simulink model "simulation_file"  (R2023b)
settings: Solver=FixedStepAuto  StartTime=0.0  StopTime=16  FixedStep=0.001  RelTol=1e-3
InitFcn:
  | importfrankaEmikaPanda
values from neighbouring files (symbols this model uses):
  d_influence = 0.06    [distance_with_linesegments_test.m]    (also in importfrankaEmikaPanda.m; matlab_obstacle_avoidance.m = 0.04)
  d_stop = 0.02    [distance_with_linesegments_test.m]    (also in importfrankaEmikaPanda.m; matlab_obstacle_avoidance.m = 0.01)
  Gripper_orientation = [-pi/4 0 0]    [importfrankaEmikaPanda.m]
  Gripper_position = [0 0 0.103399]    [importfrankaEmikaPanda.m]
  Homejointpositions = [0 ,0, 0, -pi/2, 0, pi/2, pi/4]    [importfrankaEmikaPanda.m]
  jointMaxValues = [2.8973, 1.7628, 2.8973, -0.0698, 2.8973, 3.7525, 2.8973]    [importfrankaEmikaPanda.m]
  jointMinValues = [-2.8973, -1.7628, -2.8973, -3.0718, -2.8973, 0.6500, -2.8973]    [importfrankaEmikaPanda.m]
  jointvelMaxValues = [2.1750 2.1750 2.1750 2.1750 2.6100 2.6100 2.6100]    [importfrankaEmikaPanda.m]
  jointvelMinValues = [-2.1750 -2.1750 -2.1750 -2.1750 -2.6100 -2.6100 -2.6100]    [importfrankaEmikaPanda.m]
  m = sqrt(det(JJt))    [computeManipulabilityJacobian.m]
  maxWaypoints = 20    [createWaypointData.m]    (also in importfrankaEmikaPanda.m)
  mdhparams = [ ... (first row only)    [importfrankaEmikaPanda.m]
  obstacle_sphere_1 = struct(     'type', OBSTACLE_SPHERE,      'center', [0, 0.20, 0.8],      'dimensions', [0.1, 0.1, 0.1],      'orientation', [1, 0, 0, 0],      'axis', 0  )    [importfrankaEmikaPanda.m]    (also in matlab_obstacle_avoidance.m = struct(     'type', OBSTACLE_SPHERE,      'center', [0.5545,)
  orientations = [0     0    0 ... (first row only)    [createWaypointData.m]    (also in importfrankaEmikaPanda.m = orientations'; matlab_obstacle_avoidance.m = orientations')
  ts = 0.01    [createWaypointData.m]    (also in importfrankaEmikaPanda.m = 0.001; matlab_obstacle_avoidance.m = 0.001)
  waypointAccels = zeros(size(waypointVels))    [createWaypointData.m]    (also in importfrankaEmikaPanda.m; matlab_obstacle_avoidance.m)
  waypoints = toolPositionHome' +              [0 0 0 ; 0 0 0 ; 0 0 0 ; 0 0 0 ; 0 0 0]'    [createWaypointData.m]    (also in importfrankaEmikaPanda.m = waypoints'; matlab_obstacle_avoidance.m = waypoints')
  waypointTimes = 0:4:16    [createWaypointData.m]    (also in importfrankaEmikaPanda.m; matlab_obstacle_avoidance.m)
  waypointVels = 0.1 *[ 0  0  0 ... (first row only)    [createWaypointData.m]    (also in importfrankaEmikaPanda.m; matlab_obstacle_avoidance.m)
  X = X + v0(1)    [plotCylinder.m]    (also in plotCylinder_foranimation.m)
  Y = Y + v0(2)    [plotCylinder.m]    (also in plotCylinder_foranimation.m)
  Z = Z + v0(3)    [plotCylinder.m]    (also in plotCylinder_foranimation.m)
undefined symbols (not defined in the file or in its folder): diff
libraries: sm_lib x98, nesl_utility x15, robotmaniplib x11, trajExampleUtils x9, robotcorelib x7
(part 1 of 4)
settings Model: Creator=shobhit  LastModifiedBy=shobhit
settings ModelReferenceCC: EnableRefExpFcnMdlSchedulingChecks=on

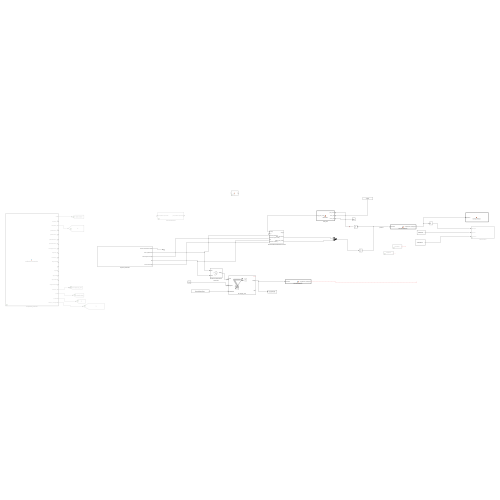
[thumbnail: Simulink's stored preview of the top-level diagram]
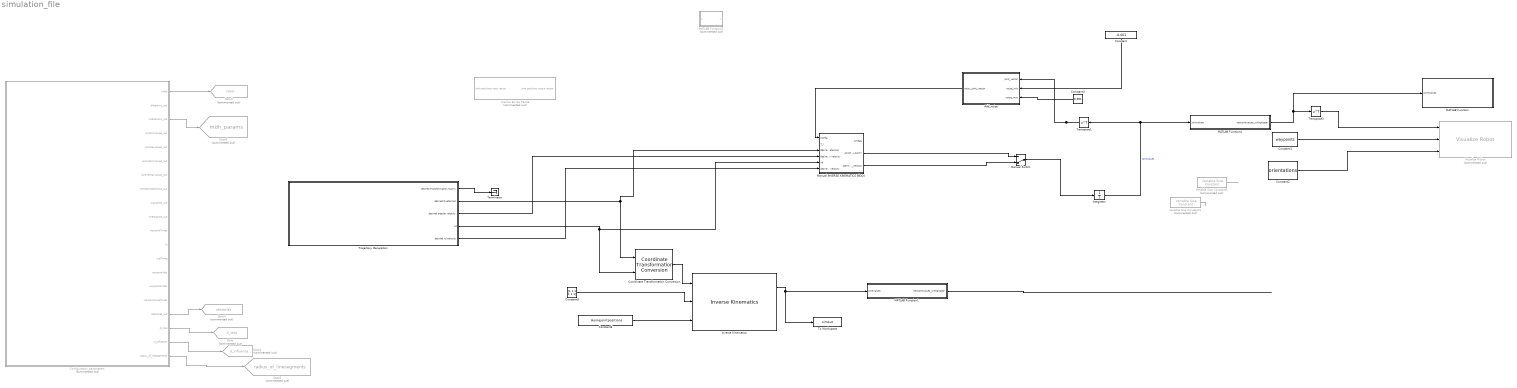
== system simulation_file ==
  Add_noise : MATLAB Function  TreatAsAtomicUnit=on
  Configuration_parameters : MATLAB Function  Commented=on  TreatAsAtomicUnit=on  SystemSampleTime=0.001
  Constant : Constant  Value=-0.001
  Constant1 : Constant  Value=waypoints  SampleTime=ts
  Constant2 : Constant  Value=orientations  VectorParams1D=off  SampleTime=ts
  Constant3 : Constant  Value=0.001
  Constant5 : Constant  Value=[1 1 1 1 1 1]
  Constant6 : Constant  Value=Homejointpositions  VectorParams1D=off
  Coordinate Transformation Conversion : robotcorelib/Coordinate Transformation Conversion  InputRepresentation=Quaternion  InputEulerSequence=ZYX  ShowTrVecInputPort=on  OutputRepresentation=Homogeneous Transformation  OutputEulerSequence=ZYX  ShowTrVecOutputPort=on  SimulateUsing=Interpreted execution
  Franka Emika Panda : Subsystem  Commented=on
  Goto : Goto  Commented=on  GotoTag=d_stop  TagVisibility=global
  Goto1 : Goto  Commented=on  GotoTag=d_influence  TagVisibility=global
  Goto2 : Goto  Commented=on  GotoTag=radius_of_linesegments  TagVisibility=global
  Goto3 : Goto  Commented=on  GotoTag=robot  TagVisibility=global
  Goto4 : Goto  Commented=on  GotoTag=obstacles  TagVisibility=global
  Goto5 : Goto  Commented=on  GotoTag=mdh_params  TagVisibility=global
  Integrator : Integrator  InitialCondition=[0 ;0; 0; -pi/2; 0; pi/2; pi/4]
  Inverse Kinematics : robotmaniplib/Inverse Kinematics  RigidBodyTree=frankarobot_mdh  EndEffector=Gripper_TCP  ShowInfo=on  SolverName=BFGS Gradient Projection  EnforceJointLimits=on  MaxIterations=1500  MaxTime=10  GradientTolerance=1e-7  SolutionTolerance=1e-6  StepTolerance=1e-14  ErrorChangeTolerance=1e-12  UseErrorDamping=on  DampingBias=0.0025  SimulateUsing=Interpreted execution
  MATLAB Function : MATLAB Function  TreatAsAtomicUnit=on
  MATLAB Function1 : MATLAB Function  TreatAsAtomicUnit=on
  MATLAB Function4 : MATLAB Function  TreatAsAtomicUnit=on
  MATLAB Function5 : MATLAB Function  Commented=on  TreatAsAtomicUnit=on
  Manual INVERSE KINEMATICS BlOCK : Subsystem
  Manual Switch : ManualSwitch  CurrentSetting=0
  Terminator : Terminator
  To Workspace : ToWorkspace  VariableName=simout  SaveFormat=Timeseries  SampleTime=-1
  Trajectory Generation : Subsystem
  Transpose1 : Math  Operator=transpose
  Transpose3 : Math  Operator=transpose
  Variable Size Constant1 : trajExampleUtils/Variable Size Constant  Commented=on  val=waypoints  maxSize=[3,maxWaypoints]  Ts=ts
  Variable Size Constant6 : trajExampleUtils/Variable Size Constant  Commented=on  val=orientations  maxSize=[3,maxWaypoints]  Ts=ts
  Visualize Robot : trajExampleUtils/Visualize Robot  Commented=on  rbtName=frankarobot  eeName=Gripper_TCP  numJoints=9  maxPts=5  plotMode=Trajectory
  wires:
  Trajectory Generation/4(xd) -> Manual INVERSE KINEMATICS BlOCK/5(xd), Coordinate Transformation Conversion/2
  Trajectory Generation/1(desired Transformation matrix) -> Terminator/1
  Variable Size Constant1/1 -> ?
  Variable Size Constant6/1 -> ?
  Constant1/1 -> Visualize Robot/2
  Constant2/1 -> Visualize Robot/3
  MATLAB Function4/1(newjointvalues_withgripper) -> MATLAB Function/1(jointValues), Transpose3/1
  Trajectory Generation/2(desired Quaternion) -> Coordinate Transformation Conversion/1, Manual INVERSE KINEMATICS BlOCK/3(desired Quaternion)
  Coordinate Transformation Conversion/1 -> Inverse Kinematics/1
  Constant5/1 -> Inverse Kinematics/2
  Constant6/1 -> Inverse Kinematics/3
  Inverse Kinematics/1 -> MATLAB Function1/1(jointvalues), To Workspace/1
  MATLAB Function1/1(newjointvalues_withgripper) -> ?
  Transpose3/1 -> Visualize Robot/1
  Integrator/1 -> Transpose1/1, MATLAB Function4/1(jointvalues)  "jointvalues"
  Trajectory Generation/3(desired angular velocity) -> Manual INVERSE KINEMATICS BlOCK/4(desired angular velocity)
  Trajectory Generation/5(desired xd velocity) -> Manual INVERSE KINEMATICS BlOCK/6(desired xd velocity)
  Manual INVERSE KINEMATICS BlOCK/2(JOINT_VELOCITY) -> Manual Switch/1
  Manual Switch/1 -> Integrator/1
  Manual INVERSE KINEMATICS BlOCK/3(optimal_joint_velocity) -> Manual Switch/2
  Constant/1 -> Add_noise/2(noise_min)
  Constant3/1 -> Add_noise/3(noise_max)
  Add_noise/1(noisy_joint_vector) -> Manual INVERSE KINEMATICS BlOCK/1(Config)
  Transpose1/1 -> Add_noise/1(joint_vector)
  Configuration_parameters/18(d_stop) -> Goto/1
  Configuration_parameters/19(d_influence) -> Goto1/1
  Configuration_parameters/20(radius_of_linesegments) -> Goto2/1
  Configuration_parameters/1(robot) -> Goto3/1
  Configuration_parameters/17(obstacles_out) -> Goto4/1
  Configuration_parameters/3(mdhparams_out) -> Goto5/1

== system simulation_file/Franka Emika Panda ==
  joint positions input vector : Inport
  Demux : Demux  Outputs=7
  Franka_Robot : Subsystem
  Joint positions vector from sensor : Mux  Inputs=7
  joint positions output vector : Outport
  wires:
  Franka_Robot/4(Output3) -> Joint positions vector from sensor/4
  Joint positions vector from sensor/1 -> joint positions output vector/1
  Franka_Robot/1(Output) -> Joint positions vector from sensor/1
  Demux/6 -> Franka_Robot/6(Input5)
  joint positions input vector/1 -> Demux/1
  Demux/5 -> Franka_Robot/5(Input4)
  Demux/3 -> Franka_Robot/3(Input2)
  Franka_Robot/6(Output5) -> Joint positions vector from sensor/6
  Demux/4 -> Franka_Robot/4(Input3)
  Demux/7 -> Franka_Robot/7(Input6)
  Franka_Robot/2(Output1) -> Joint positions vector from sensor/2
  Franka_Robot/3(Output2) -> Joint positions vector from sensor/3
  Demux/1 -> Franka_Robot/1(Input)
  Franka_Robot/7(Output6) -> Joint positions vector from sensor/7
  Demux/2 -> Franka_Robot/2(Input1)
  Franka_Robot/5(Output4) -> Joint positions vector from sensor/5

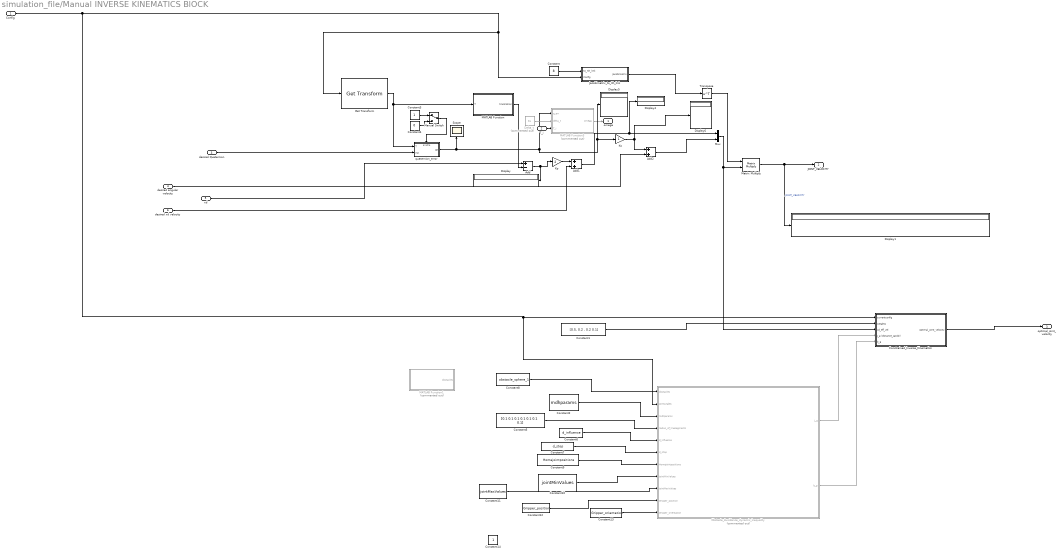
== system simulation_file/Manual INVERSE KINEMATICS BlOCK ==
  Config : Inport
  T_i : Inport  Port=2
  desired Quaternion : Inport  Port=3
  desired angular velocity : Inport  Port=4
  xd : Inport  Port=5
  desired xd velocity : Inport  Port=6
  Add : Sum  Inputs=+-
  Add1 : Sum
  Add2 : Sum
  Constant : Constant  Value=8
  Constant1 : Constant  Value=[0.5, 0.2 , 0.2 0.1]
  Constant10 : Constant  Value=jointMinValues  VectorParams1D=off
  Constant11 : Constant  Value=jointMaxValues  VectorParams1D=off
  Constant12 : Constant  Value=Gripper_position  VectorParams1D=off
  Constant13 : Constant  Value=Gripper_orientation  VectorParams1D=off
  Constant14 : Constant
  Constant2 : Constant  Value=mdhparams  VectorParams1D=off
  Constant3 : Constant
  Constant4 : Constant  Value=0
  Constant5 : Constant  Value=[0.1 0.1 0.1 0.1 0.1 0.1 0.1]  VectorParams1D=off
  Constant6 : Constant  Value=d_influence  VectorParams1D=off
  Constant7 : Constant  Value=d_stop  VectorParams1D=off
  Constant8 : Constant  Value=obstacle_sphere_1  VectorParams1D=off  OutDataTypeStr=Bus: slBus1
  Constant9 : Constant  Value=Homejointpositions  VectorParams1D=off
  Constrained_Inverse_Kinematics : Subsystem
  Delta_t : Constant  Commented=on  Value=ts
  Display{,1,4..6} (5 alike) : Display
  Get Transform : robotmaniplib/Get Transform  RigidBodyTree=frankarobot_mdh  SourceBody=Gripper_TCP  TargetBody=base  SimulateUsing=Interpreted execution
  Jacobimatrix_to_ith_link : Subsystem
  Ko : Gain
  Kp : Gain  Gain=2
  MATLAB Function : MATLAB Function  TreatAsAtomicUnit=on
  MATLAB Function1 : MATLAB Function  Commented=on  TreatAsAtomicUnit=on
  MATLAB Function3 : MATLAB Function  Commented=on  TreatAsAtomicUnit=on
  Manual Switch : ManualSwitch
  Matrix Multiply : Product  Multiplication=Matrix(*)
  Mux : Mux  Inputs=2
  Obstacle_Avoidance_dynamic_inequality : MATLAB Function  Commented=on  TreatAsAtomicUnit=on
  Scope : Scope
  Transpose : Math  Operator=transpose
  quaternion_error : Subsystem
  omega : Outport
  JOINT_VELOCITY : Outport  Port=2
  optimal_joint_velocity : Outport  Port=3
  wires:
  MATLAB Function/1(translation) -> Add/2
  desired Quaternion/1 -> quaternion_error/2(In2)
  Manual Switch/1 -> quaternion_error/Enable
  MATLAB Function3/1(omega) -> omega/1
  Kp/1 -> Add1/1
  quaternion_error/1(qe) -> Ko/1, Display5/1, MATLAB Function3/1(q_err), Scope/1
  Add/1 -> Display/1, Kp/1
  Mux/1 -> Constrained_Inverse_Kinematics/3(xd_eff_vel), Matrix Multiply/2
  Constant4/1 -> Manual Switch/2
  Constant3/1 -> Manual Switch/1
  Ko/1 -> Display6/1, Add2/1
  Add2/1 -> Mux/2
  Jacobimatrix_to_ith_link/1(Jacobimatrix) -> Transpose/1
  Matrix Multiply/1 -> JOINT_VELOCITY/1, Display1/1  "JOINT_VELOCITY"
  Get Transform/1 -> quaternion_error/1(T), MATLAB Function/1(T)
  desired angular velocity/1 -> Add2/2
  xd/1 -> Add/1
  Constant/1 -> Jacobimatrix_to_ith_link/1(to_ith_link)
  desired xd velocity/1 -> Add1/2
  Transpose/1 -> Matrix Multiply/1
  Add1/1 -> Display4/1, Mux/1
  T_i/1 -> MATLAB Function3/3(T_i)
  Delta_t/1 -> MATLAB Function3/2(delta_t)
  Constant1/1 -> Constrained_Inverse_Kinematics/2(weights)
  Config/1 -> Obstacle_Avoidance_dynamic_inequality/2(jointAngles), Constrained_Inverse_Kinematics/1(currentconfig), Jacobimatrix_to_ith_link/2(Config), Get Transform/1
  Constrained_Inverse_Kinematics/1(optimal_joint_velocity) -> optimal_joint_velocity/1
  Obstacle_Avoidance_dynamic_inequality/1(J_g) -> Constrained_Inverse_Kinematics/4(J_g (distance_Jacobi))
  Obstacle_Avoidance_dynamic_inequality/2(b_g) -> Constrained_Inverse_Kinematics/5("b_g ")
  Constant2/1 -> Obstacle_Avoidance_dynamic_inequality/3(mdhparams)
  Constant5/1 -> Obstacle_Avoidance_dynamic_inequality/4(radius_of_linesegments)
  Constant6/1 -> Obstacle_Avoidance_dynamic_inequality/5(d_influence)
  Constant7/1 -> Obstacle_Avoidance_dynamic_inequality/6(d_stop)
  Constant8/1 -> Obstacle_Avoidance_dynamic_inequality/1(obstacles)
  Constant9/1 -> Obstacle_Avoidance_dynamic_inequality/7(Homejointpositions)
  Constant10/1 -> Obstacle_Avoidance_dynamic_inequality/8(jointMinValues)
  Constant11/1 -> Obstacle_Avoidance_dynamic_inequality/9(jointMaxValues)
  Constant12/1 -> Obstacle_Avoidance_dynamic_inequality/10(Gripper_position)
  Constant13/1 -> Obstacle_Avoidance_dynamic_inequality/11(Gripper_orientation)

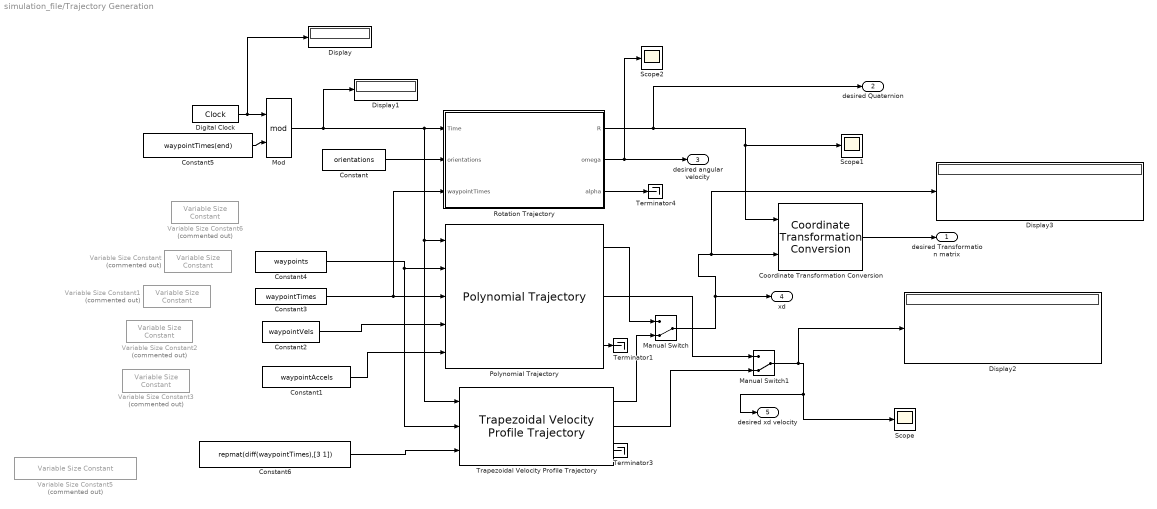
== system simulation_file/Trajectory Generation ==
  Constant : Constant  Value=orientations  SampleTime=ts
  Constant1 : Constant  Value=waypointAccels  SampleTime=ts
  Constant2 : Constant  Value=waypointVels  SampleTime=ts
  Constant3 : Constant  Value=waypointTimes  SampleTime=ts
  Constant4 : Constant  Value=waypoints  SampleTime=ts
  Constant5 : Constant  Value=waypointTimes(end)
  Constant6 : Constant  Value=repmat(diff(waypointTimes),[3 1])  SampleTime=ts
  Coordinate Transformation Conversion : robotcorelib/Coordinate Transformation Conversion  InputRepresentation=Quaternion  InputEulerSequence=ZYX  ShowTrVecInputPort=on  OutputRepresentation=Homogeneous Transformation  OutputEulerSequence=ZYX  ShowTrVecOutputPort=on  SimulateUsing=Interpreted execution
  Digital Clock : DigitalClock  SampleTime=ts
  Display{,1..3} (4 alike) : Display
  Manual Switch : ManualSwitch  CurrentSetting=0
  Manual Switch1 : ManualSwitch  CurrentSetting=0
  Mod : Math  Operator=mod  SignedPower=on
  Polynomial Trajectory : robotcorelib/Polynomial Trajectory  WaypointSource=External  Waypoints=[ 0, 2, 1, 5, 0; -1, 3, 1, 4, 4 ]  TimePoints=[ 0, 1, 2, 3, 4 ]  TimeInterval=[ 1, 4 ]  Method=Quintic Polynomial  ParameterSource=External  VelocityBoundaryCondition=zeros( 2, 5 )  AccelerationBoundaryCondition=zeros( 2, 5 )  SimulateUsing=Interpreted execution
  Rotation Trajectory : Subsystem
  Scope : Scope
  Scope1 : Scope
  Scope2 : Scope
  Terminator1 : Terminator
  Terminator3 : Terminator
  Terminator4 : Terminator
  Trapezoidal Velocity Profile Trajectory : robotcorelib/Trapezoidal Velocity Profile Trajectory  WaypointSource=External  Waypoints=[ 0, -0.5, -1; 0, 0.5, 1 ]  NumParams=1  Parameter1=End Time  Parameter2=End Time  ParameterSource=External  PeakVelocity=[ 1; 1; 1 ]  Acceleration=[ 1; 2 ]  EndTime=[ 1; 1; 1 ]  AccelTime=[ 1; 2 ]  SimulateUsing=Interpreted execution
  Variable Size Constant : trajExampleUtils/Variable Size Constant  Commented=on  val=waypoints  maxSize=[3,maxWaypoints]  Ts=ts
  Variable Size Constant1 : trajExampleUtils/Variable Size Constant  Commented=on  val=waypointTimes  maxSize=[1,maxWaypoints]  Ts=ts
  Variable Size Constant2 : trajExampleUtils/Variable Size Constant  Commented=on  val=waypointVels  maxSize=[3,maxWaypoints]  Ts=ts
  Variable Size Constant3 : trajExampleUtils/Variable Size Constant  Commented=on  val=waypointAccels  maxSize=[3,maxWaypoints]  Ts=ts
  Variable Size Constant5 : trajExampleUtils/Variable Size Constant  Commented=on  val=repmat(diff(waypointTimes),[3 1])  maxSize=[3,maxWaypoints-1]  Ts=ts
  Variable Size Constant6 : trajExampleUtils/Variable Size Constant  Commented=on  val=orientations  maxSize=[3,maxWaypoints]  Ts=ts
  desired Transformation matrix : Outport
  desired Quaternion : Outport  Port=2
  desired angular velocity : Outport  Port=3
  xd : Outport  Port=4
  desired xd velocity : Outport  Port=5
  wires:
  Trapezoidal Velocity Profile Trajectory/3 -> Terminator3/1
  Constant2/1 -> Polynomial Trajectory/4
  Constant4/1 -> Trapezoidal Velocity Profile Trajectory/2, Polynomial Trajectory/2
  Constant6/1 -> Trapezoidal Velocity Profile Trajectory/3
  Polynomial Trajectory/3 -> Terminator1/1
  Polynomial Trajectory/1 -> Manual Switch/1
  Trapezoidal Velocity Profile Trajectory/1 -> Manual Switch/2
  Constant/1 -> Rotation Trajectory/2(orientations)
  Trapezoidal Velocity Profile Trajectory/2 -> Manual Switch1/2
  Mod/1 -> Display1/1, Rotation Trajectory/1(Time), Trapezoidal Velocity Profile Trajectory/1, Polynomial Trajectory/1
  Constant1/1 -> Polynomial Trajectory/5
  Coordinate Transformation Conversion/1 -> desired Transformation matrix/1
  Constant3/1 -> Rotation Trajectory/3(waypointTimes), Polynomial Trajectory/3
  Rotation Trajectory/1(R) -> desired Quaternion/1, Coordinate Transformation Conversion/1, Scope1/1
  Constant5/1 -> Mod/2
  Digital Clock/1 -> Display/1, Mod/1
  Polynomial Trajectory/2 -> Manual Switch1/1
  Manual Switch/1 -> Display3/1, Coordinate Transformation Conversion/2, xd/1
  Rotation Trajectory/2(omega) -> Scope2/1, desired angular velocity/1
  Rotation Trajectory/3(alpha) -> Terminator4/1
  Manual Switch1/1 -> Display2/1, Scope/1, desired xd velocity/1

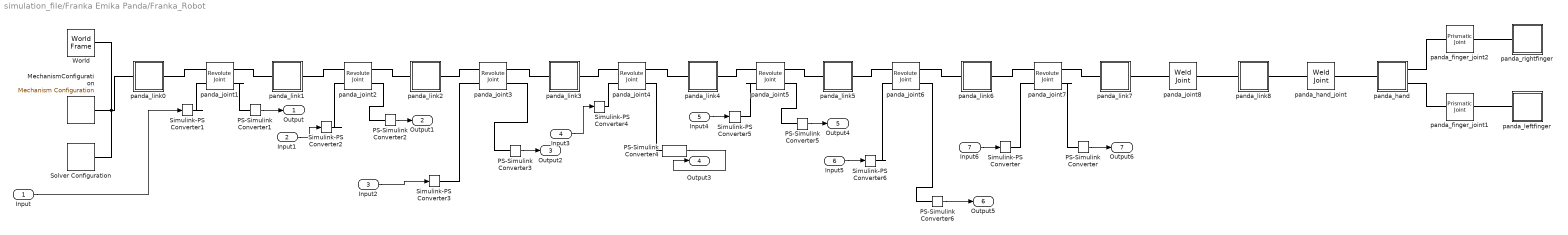
== system simulation_file/Franka Emika Panda/Franka_Robot ==
  Input : Inport
  Input1 : Inport  Port=2
  Input2 : Inport  Port=3
  Input3 : Inport  Port=4
  Input4 : Inport  Port=5
  Input5 : Inport  Port=6
  Input6 : Inport  Port=7
  MechanismConfiguration : sm_lib/Utilities/Mechanism Configuration  UniformGravity=Constant  GravityVector=[0, 0, 0]  GravityVectorUnits=m/s^2  LinearizationDelta=0.001  JointModeTransitionNonlinearIterations=2
  PS-Simulink Converter{,1..6} (7 alike) : nesl_utility/PS-Simulink Converter  PhysicalDomain=network_engine_domain  SubClassName=ps_output  LeftPortType=input  RightPortType=output  PseudoPeriodic=off  Frequencies=[]  VectorFormat=inherit  Unit=inherit  AffineConversion=off
  Simulink-PS Converter{,1,3..6} (6 alike) : nesl_utility/Simulink-PS Converter  PhysicalDomain=network_engine_domain  SubClassName=ps_input  LeftPortType=input  RightPortType=output  PseudoPeriodic=off  Frequencies=[]  NoiseDistribution=none  NoiseParameters=[]  Unit=1  AffineConversion=off  FilteringAndDerivatives=provide  SimscapeFilterOrder=1  InputFilterTimeConstant=0.001  UdotUserProvided=0
  Simulink-PS Converter2 : nesl_utility/Simulink-PS Converter  PhysicalDomain=network_engine_domain  SubClassName=ps_input  LeftPortType=input  RightPortType=output  PseudoPeriodic=off  Frequencies=[]  NoiseDistribution=none  NoiseParameters=[]  Unit=1  AffineConversion=off  FilteringAndDerivatives=filter  SimscapeFilterOrder=1  InputFilterTimeConstant=0.001  UdotUserProvided=0
  Solver Configuration : nesl_utility/Solver Configuration  PhysicalDomain=network_engine_domain  SubClassName=solver  LeftPortType=input  RightPortType=generic  Tones=[]  Harmonics=[]  SimulateNoise=off  Profile=off  UseLocalSampling=off  EnableSwitchedLinearOptims=on  FrequencyDomain=off  UseCCode=off  RelTol=0.001  AbsTol=0.001  MinStep=1e-09  ToWorkspace=off  RevertToSquareIcSolve=off  NumHomotopyIterations=100  PhasorMode=off  PhasorModeNumHarmonics=1  ConsistencySolver=NEWTON_XTOL_AFTER_FTOL  IndexReductionMethod=DerivativeReplacement  DoDC=off  ResidualTolerance=1e-09  ConsistencyTolSource=GLOBAL  ConsistencyAbsTol=0.001  ConsistencyRelTol=0.001  ConsistencyTolFactor=0.001  UseLocalSolver=off  LocalSolverChoice=NE_BACKWARD_EULER_ADVANCER  ResolveIndetEquations=on  FunctionEvalNumThread=1  LocalSolverSampleTime=0.001  DoFixedCost=off  MaxNonlinIter=3  MaxModeIter=2  ComputeImpulses=off  ImpulseIterations=2  LinearAlgebra=auto  LinearAlgebraNumThread=0  EquationFormulation=NE_TIME_EF  DelaysMemoryBudget=1024  AutomaticFiltering=on  FilteringTimeConstant=0.001  PartitionStorageMethod=AS_NEEDED  PartitionMemoryBudget=1024  PartitionMethod=ROBUST  MultibodyUseLocalSolver=off  MultibodyLocalSolverChoice=ODE1  MultibodyLocalSolverSampleTime=0.001
  World : sm_lib/Frames and Transforms/World Frame
  panda_finger_joint1 : sm_lib/Joints/Prismatic Joint  JointMode=Normal  SenseConstraintForce=off  SenseConstraintForceX=off  SenseConstraintForceY=off  SenseConstraintForceZ=off  SenseConstraintTorque=off  SenseConstraintTorqueX=off  SenseConstraintTorqueY=off  SenseConstraintTorqueZ=off  SenseTotalForce=off  SenseTotalForceX=off  SenseTotalForceY=off  SenseTotalForceZ=off  SenseTotalTorque=off  SenseTotalTorqueX=off  SenseTotalTorqueY=off  SenseTotalTorqueZ=off  CompositeWrenchDir=FollowerOnBase  CompositeWrenchFrame=BaseFrame  EquilibriumPosition=0  EquilibriumPositionUnits=m  SpringStiffness=0  SpringStiffnessUnits=N/m  DampingCoefficient=0  DampingCoefficientUnits=kg/s  TorqueActuationMode=NoTorque  MotionActuationMode=ComputedMotion  SensePosition=off  SenseVelocity=off  SenseAcceleration=off  SenseTorqueForce=off  SenseLowerLimitTorqueForce=off  SenseUpperLimitTorqueForce=off  LowerLimitSpecify=on  LowerLimitBound=0  LowerLimitBoundUnits=m  LowerLimitStiffness=1e6  LowerLimitStiffnessUnits=N/m  LowerLimitDamping=1e3  LowerLimitDampingUnits=N/(m/s)  LowerLimitTransitionRegionWidth=1e-4  LowerLimitTransitionRegionWidthUnits=m  UpperLimitSpecify=on  UpperLimitBound=0.04  UpperLimitBoundUnits=m  UpperLimitStiffness=1e6  UpperLimitStiffnessUnits=N/m  UpperLimitDamping=1e3  UpperLimitDampingUnits=N/(m/s)  UpperLimitTransitionRegionWidth=1e-4  UpperLimitTransitionRegionWidthUnits=m  PositionTargetSpecify=on  PositionTargetPriority=High  PositionTargetValue=0  PositionTargetValueUnits=m  VelocityTargetSpecify=off  VelocityTargetPriority=High  VelocityTargetValue=0  VelocityTargetValueUnits=m/s
  panda_finger_joint2 : sm_lib/Joints/Prismatic Joint  JointMode=Normal  SenseConstraintForce=off  SenseConstraintForceX=off  SenseConstraintForceY=off  SenseConstraintForceZ=off  SenseConstraintTorque=off  SenseConstraintTorqueX=off  SenseConstraintTorqueY=off  SenseConstraintTorqueZ=off  SenseTotalForce=off  SenseTotalForceX=off  SenseTotalForceY=off  SenseTotalForceZ=off  SenseTotalTorque=off  SenseTotalTorqueX=off  SenseTotalTorqueY=off  SenseTotalTorqueZ=off  CompositeWrenchDir=FollowerOnBase  CompositeWrenchFrame=BaseFrame  EquilibriumPosition=0  EquilibriumPositionUnits=m  SpringStiffness=0  SpringStiffnessUnits=N/m  DampingCoefficient=0  DampingCoefficientUnits=kg/s  TorqueActuationMode=NoTorque  MotionActuationMode=ComputedMotion  SensePosition=off  SenseVelocity=off  SenseAcceleration=off  SenseTorqueForce=off  SenseLowerLimitTorqueForce=off  SenseUpperLimitTorqueForce=off  LowerLimitSpecify=on  LowerLimitBound=0  LowerLimitBoundUnits=m  LowerLimitStiffness=1e6  LowerLimitStiffnessUnits=N/m  LowerLimitDamping=1e3  LowerLimitDampingUnits=N/(m/s)  LowerLimitTransitionRegionWidth=1e-4  LowerLimitTransitionRegionWidthUnits=m  UpperLimitSpecify=on  UpperLimitBound=0.04  UpperLimitBoundUnits=m  UpperLimitStiffness=1e6  UpperLimitStiffnessUnits=N/m  UpperLimitDamping=1e3  UpperLimitDampingUnits=N/(m/s)  UpperLimitTransitionRegionWidth=1e-4  UpperLimitTransitionRegionWidthUnits=m  PositionTargetSpecify=on  PositionTargetPriority=High  PositionTargetValue=0  PositionTargetValueUnits=m  VelocityTargetSpecify=off  VelocityTargetPriority=High  VelocityTargetValue=0  VelocityTargetValueUnits=m/s
  panda_hand : Subsystem
  panda_hand_joint : sm_lib/Joints/Weld Joint  JointMode=Normal  SenseConstraintForce=off  SenseConstraintForceX=off  SenseConstraintForceY=off  SenseConstraintForceZ=off  SenseConstraintTorque=off  SenseConstraintTorqueX=off  SenseConstraintTorqueY=off  SenseConstraintTorqueZ=off  SenseTotalForce=off  SenseTotalForceX=off  SenseTotalForceY=off  SenseTotalForceZ=off  SenseTotalTorque=off  SenseTotalTorqueX=off  SenseTotalTorqueY=off  SenseTotalTorqueZ=off  CompositeWrenchDir=FollowerOnBase  CompositeWrenchFrame=BaseFrame
  panda_joint{1,3,5,7} (4 alike) : sm_lib/Joints/Revolute Joint  JointMode=Normal  SenseConstraintForce=off  SenseConstraintForceX=off  SenseConstraintForceY=off  SenseConstraintForceZ=off  SenseConstraintTorque=off  SenseConstraintTorqueX=off  SenseConstraintTorqueY=off  SenseConstraintTorqueZ=off  SenseTotalForce=off  SenseTotalForceX=off  SenseTotalForceY=off  SenseTotalForceZ=off  SenseTotalTorque=off  SenseTotalTorqueX=off  SenseTotalTorqueY=off  SenseTotalTorqueZ=off  CompositeWrenchDir=FollowerOnBase  CompositeWrenchFrame=BaseFrame  EquilibriumPosition=0  EquilibriumPositionUnits=deg  SpringStiffness=0  SpringStiffnessUnits=N*m/deg  DampingCoefficient=0  DampingCoefficientUnits=kg*m^2/(rad*s)  TorqueActuationMode=NoTorque  MotionActuationMode=InputMotion  SensePosition=on  SenseVelocity=off  SenseAcceleration=off  SenseTorqueForce=off  SenseLowerLimitTorqueForce=off  SenseUpperLimitTorqueForce=off  LowerLimitSpecify=on  LowerLimitBound=-2.8973  LowerLimitBoundUnits=rad  LowerLimitStiffness=1e4  LowerLimitStiffnessUnits=N*m/deg  LowerLimitDamping=10  LowerLimitDampingUnits=N*m/(deg/s)  LowerLimitTransitionRegionWidth=0.1  LowerLimitTransitionRegionWidthUnits=deg  UpperLimitSpecify=on  UpperLimitBound=2.8973  UpperLimitBoundUnits=rad  UpperLimitStiffness=1e4  UpperLimitStiffnessUnits=N*m/deg  UpperLimitDamping=10  UpperLimitDampingUnits=N*m/(deg/s)  UpperLimitTransitionRegionWidth=0.1  UpperLimitTransitionRegionWidthUnits=deg  PositionTargetSpecify=off  PositionTargetPriority=High  PositionTargetValue=0  PositionTargetValueUnits=rad  VelocityTargetSpecify=off  VelocityTargetPriority=High  VelocityTargetValue=0  VelocityTargetValueUnits=deg/s
  panda_joint2 : sm_lib/Joints/Revolute Joint  JointMode=Normal  SenseConstraintForce=off  SenseConstraintForceX=off  SenseConstraintForceY=off  SenseConstraintForceZ=off  SenseConstraintTorque=off  SenseConstraintTorqueX=off  SenseConstraintTorqueY=off  SenseConstraintTorqueZ=off  SenseTotalForce=off  SenseTotalForceX=off  SenseTotalForceY=off  SenseTotalForceZ=off  SenseTotalTorque=off  SenseTotalTorqueX=off  SenseTotalTorqueY=off  SenseTotalTorqueZ=off  CompositeWrenchDir=FollowerOnBase  CompositeWrenchFrame=BaseFrame  EquilibriumPosition=0  EquilibriumPositionUnits=deg  SpringStiffness=0  SpringStiffnessUnits=N*m/deg  DampingCoefficient=0  DampingCoefficientUnits=kg*m^2/(rad*s)  TorqueActuationMode=NoTorque  MotionActuationMode=InputMotion  SensePosition=on  SenseVelocity=off  SenseAcceleration=off  SenseTorqueForce=off  SenseLowerLimitTorqueForce=off  SenseUpperLimitTorqueForce=off  LowerLimitSpecify=on  LowerLimitBound=-1.7628  LowerLimitBoundUnits=rad  LowerLimitStiffness=1e4  LowerLimitStiffnessUnits=N*m/deg  LowerLimitDamping=10  LowerLimitDampingUnits=N*m/(deg/s)  LowerLimitTransitionRegionWidth=0.1  LowerLimitTransitionRegionWidthUnits=deg  UpperLimitSpecify=on  UpperLimitBound=1.7628  UpperLimitBoundUnits=rad  UpperLimitStiffness=1e4  UpperLimitStiffnessUnits=N*m/deg  UpperLimitDamping=10  UpperLimitDampingUnits=N*m/(deg/s)  UpperLimitTransitionRegionWidth=0.1  UpperLimitTransitionRegionWidthUnits=deg  PositionTargetSpecify=off  PositionTargetPriority=High  PositionTargetValue=-1.5708  PositionTargetValueUnits=rad  VelocityTargetSpecify=off  VelocityTargetPriority=High  VelocityTargetValue=0  VelocityTargetValueUnits=deg/s
  panda_joint4 : sm_lib/Joints/Revolute Joint  JointMode=Normal  SenseConstraintForce=off  SenseConstraintForceX=off  SenseConstraintForceY=off  SenseConstraintForceZ=off  SenseConstraintTorque=off  SenseConstraintTorqueX=off  SenseConstraintTorqueY=off  SenseConstraintTorqueZ=off  SenseTotalForce=off  SenseTotalForceX=off  SenseTotalForceY=off  SenseTotalForceZ=off  SenseTotalTorque=off  SenseTotalTorqueX=off  SenseTotalTorqueY=off  SenseTotalTorqueZ=off  CompositeWrenchDir=FollowerOnBase  CompositeWrenchFrame=BaseFrame  EquilibriumPosition=0  EquilibriumPositionUnits=deg  SpringStiffness=0  SpringStiffnessUnits=N*m/deg  DampingCoefficient=0  DampingCoefficientUnits=kg*m^2/(rad*s)  TorqueActuationMode=NoTorque  MotionActuationMode=InputMotion  SensePosition=on  SenseVelocity=off  SenseAcceleration=off  SenseTorqueForce=off  SenseLowerLimitTorqueForce=off  SenseUpperLimitTorqueForce=off  LowerLimitSpecify=on  LowerLimitBound=-3.0718  LowerLimitBoundUnits=rad  LowerLimitStiffness=1e4  LowerLimitStiffnessUnits=N*m/deg  LowerLimitDamping=10  LowerLimitDampingUnits=N*m/(deg/s)  LowerLimitTransitionRegionWidth=0.1  LowerLimitTransitionRegionWidthUnits=deg  UpperLimitSpecify=on  UpperLimitBound=-0.0698  UpperLimitBoundUnits=rad  UpperLimitStiffness=1e4  UpperLimitStiffnessUnits=N*m/deg  UpperLimitDamping=10  UpperLimitDampingUnits=N*m/(deg/s)  UpperLimitTransitionRegionWidth=0.1  UpperLimitTransitionRegionWidthUnits=deg  PositionTargetSpecify=off  PositionTargetPriority=High  PositionTargetValue=0  PositionTargetValueUnits=rad  VelocityTargetSpecify=off  VelocityTargetPriority=High  VelocityTargetValue=0  VelocityTargetValueUnits=deg/s
  panda_joint6 : sm_lib/Joints/Revolute Joint  JointMode=Normal  SenseConstraintForce=off  SenseConstraintForceX=off  SenseConstraintForceY=off  SenseConstraintForceZ=off  SenseConstraintTorque=off  SenseConstraintTorqueX=off  SenseConstraintTorqueY=off  SenseConstraintTorqueZ=off  SenseTotalForce=off  SenseTotalForceX=off  SenseTotalForceY=off  SenseTotalForceZ=off  SenseTotalTorque=off  SenseTotalTorqueX=off  SenseTotalTorqueY=off  SenseTotalTorqueZ=off  CompositeWrenchDir=FollowerOnBase  CompositeWrenchFrame=BaseFrame  EquilibriumPosition=0  EquilibriumPositionUnits=deg  SpringStiffness=0  SpringStiffnessUnits=N*m/deg  DampingCoefficient=0  DampingCoefficientUnits=kg*m^2/(rad*s)  TorqueActuationMode=NoTorque  MotionActuationMode=InputMotion  SensePosition=on  SenseVelocity=off  SenseAcceleration=off  SenseTorqueForce=off  SenseLowerLimitTorqueForce=off  SenseUpperLimitTorqueForce=off  LowerLimitSpecify=on  LowerLimitBound=-0.0175  LowerLimitBoundUnits=rad  LowerLimitStiffness=1e4  LowerLimitStiffnessUnits=N*m/deg  LowerLimitDamping=10  LowerLimitDampingUnits=N*m/(deg/s)  LowerLimitTransitionRegionWidth=0.1  LowerLimitTransitionRegionWidthUnits=deg  UpperLimitSpecify=on  UpperLimitBound=3.7525  UpperLimitBoundUnits=rad  UpperLimitStiffness=1e4  UpperLimitStiffnessUnits=N*m/deg  UpperLimitDamping=10  UpperLimitDampingUnits=N*m/(deg/s)  UpperLimitTransitionRegionWidth=0.1  UpperLimitTransitionRegionWidthUnits=deg  PositionTargetSpecify=off  PositionTargetPriority=High  PositionTargetValue=0  PositionTargetValueUnits=rad  VelocityTargetSpecify=off  VelocityTargetPriority=High  VelocityTargetValue=0  VelocityTargetValueUnits=deg/s
  panda_joint8 : sm_lib/Joints/Weld Joint  JointMode=Normal  SenseConstraintForce=off  SenseConstraintForceX=off  SenseConstraintForceY=off  SenseConstraintForceZ=off  SenseConstraintTorque=off  SenseConstraintTorqueX=off  SenseConstraintTorqueY=off  SenseConstraintTorqueZ=off  SenseTotalForce=off  SenseTotalForceX=off  SenseTotalForceY=off  SenseTotalForceZ=off  SenseTotalTorque=off  SenseTotalTorqueX=off  SenseTotalTorqueY=off  SenseTotalTorqueZ=off  CompositeWrenchDir=FollowerOnBase  CompositeWrenchFrame=BaseFrame
  panda_leftfinger : Subsystem
  panda_link0 : Subsystem
  panda_link1 : Subsystem
  panda_link2 : Subsystem
  panda_link3 : Subsystem
  panda_link4 : Subsystem
  panda_link5 : Subsystem
  panda_link6 : Subsystem
  panda_link7 : Subsystem
  panda_link8 : Subsystem
  panda_rightfinger : Subsystem
  Output : Outport
  Output1 : Outport  Port=2
  Output2 : Outport  Port=3
  Output3 : Outport  Port=4
  Output4 : Outport  Port=5
  Output5 : Outport  Port=6
  Output6 : Outport  Port=7
  wires:
  Input4/1 -> Simulink-PS Converter5/1
  Input2/1 -> Simulink-PS Converter3/1
  PS-Simulink Converter6/1 -> Output5/1
  PS-Simulink Converter3/1 -> Output2/1
  Input/1 -> Simulink-PS Converter1/1
  Input1/1 -> Simulink-PS Converter2/1
  PS-Simulink Converter1/1 -> Output/1
  Input6/1 -> Simulink-PS Converter/1
  PS-Simulink Converter5/1 -> Output4/1
  PS-Simulink Converter4/1 -> Output3/1
  Input5/1 -> Simulink-PS Converter6/1
  PS-Simulink Converter/1 -> Output6/1
  PS-Simulink Converter2/1 -> Output1/1
  Input3/1 -> Simulink-PS Converter4/1
  connections:
  PS-Simulink Converter6/LConn1 -- panda_joint6/RConn2
  Simulink-PS Converter1/RConn1 -- panda_joint1/LConn2
  panda_joint3/LConn2 -- Simulink-PS Converter3/RConn1
  PS-Simulink Converter2/LConn1 -- panda_joint2/RConn2
  panda_joint8/LConn1 -- panda_link7/RConn1
  panda_joint7/RConn2 -- PS-Simulink Converter/LConn1
  panda_joint4/LConn2 -- Simulink-PS Converter4/RConn1
  panda_finger_joint2/LConn1 -- panda_hand/RConn1
  panda_joint3/RConn2 -- PS-Simulink Converter3/LConn1
  panda_joint6/LConn1 -- panda_link5/RConn1
  panda_finger_joint1/RConn1 -- panda_leftfinger/LConn1
  panda_hand/LConn1 -- panda_hand_joint/RConn1
  panda_finger_joint2/RConn1 -- panda_rightfinger/LConn1
  panda_joint8/RConn1 -- panda_link8/LConn1
  Simulink-PS Converter/RConn1 -- panda_joint7/LConn2
  panda_joint3/RConn1 -- panda_link3/LConn1
  Simulink-PS Converter6/RConn1 -- panda_joint6/LConn2
  panda_joint7/LConn1 -- panda_link6/RConn1
  panda_joint4/RConn1 -- panda_link4/LConn1
  panda_joint5/RConn1 -- panda_link5/LConn1
  panda_joint1/RConn1 -- panda_link1/LConn1
  panda_finger_joint1/LConn1 -- panda_hand/RConn2
  World/RConn1 -- MechanismConfiguration/RConn1 -- Solver Configuration/RConn1 -- panda_link0/LConn1
  panda_joint3/LConn1 -- panda_link2/RConn1
  panda_hand_joint/LConn1 -- panda_link8/RConn1
  panda_joint5/LConn2 -- Simulink-PS Converter5/RConn1
  panda_joint4/RConn2 -- PS-Simulink Converter4/LConn1
  panda_joint2/RConn1 -- panda_link2/LConn1
  panda_joint7/RConn1 -- panda_link7/LConn1
  panda_joint6/RConn1 -- panda_link6/LConn1
  panda_joint2/LConn1 -- panda_link1/RConn1
  panda_joint4/LConn1 -- panda_link3/RConn1
  panda_joint1/RConn2 -- PS-Simulink Converter1/LConn1
  panda_joint1/LConn1 -- panda_link0/RConn1
  PS-Simulink Converter5/LConn1 -- panda_joint5/RConn2
  panda_joint5/LConn1 -- panda_link4/RConn1
  Simulink-PS Converter2/RConn1 -- panda_joint2/LConn2

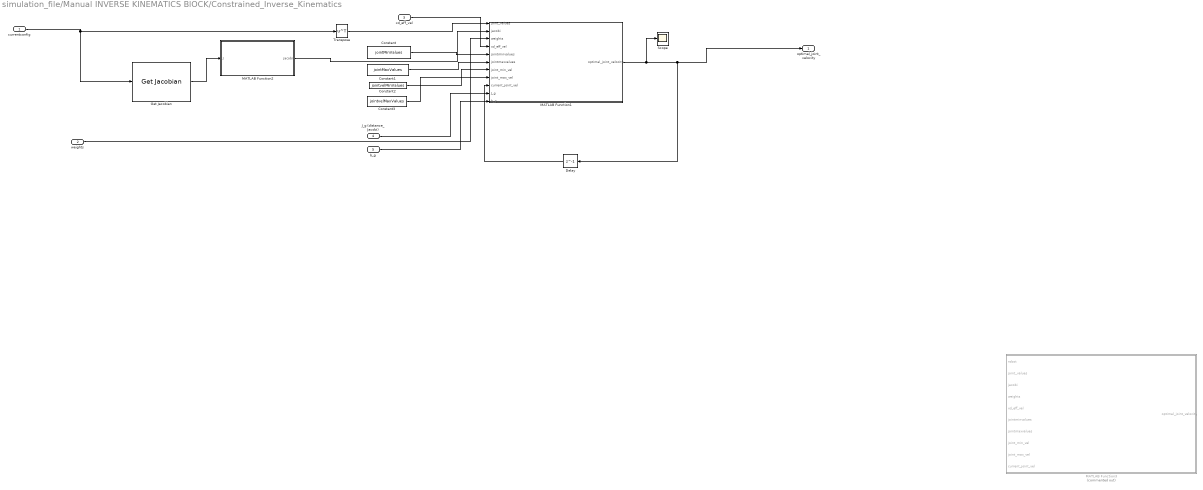
== system simulation_file/Manual INVERSE KINEMATICS BlOCK/Constrained_Inverse_Kinematics ==
  currentconfig : Inport
  weights : Inport  Port=2
  xd_eff_vel : Inport  Port=3
  J_g (distance_Jacobi) : Inport  Port=4
  "b_g " : Inport  Port=5
  Constant : Constant  Value=jointMinValues  VectorParams1D=off
  Constant1 : Constant  Value=jointMaxValues  VectorParams1D=off
  Constant2 : Constant  Value=jointvelMinValues  VectorParams1D=off
  Constant3 : Constant  Value=jointvelMaxValues  VectorParams1D=off
  Delay : Delay  DelayLength=1
  Get Jacobian : robotmaniplib/Get Jacobian  RigidBodyTree=frankarobot_mdh  EndEffector=Gripper_TCP  SimulateUsing=Interpreted execution
  MATLAB Function1 : MATLAB Function  TreatAsAtomicUnit=on
  MATLAB Function2 : MATLAB Function  TreatAsAtomicUnit=on
  MATLAB Function3 : MATLAB Function  Commented=on  TreatAsAtomicUnit=on
  Scope : Scope
  Transpose : Math  Operator=transpose
  optimal_joint_velocity : Outport
  wires:
  Get Jacobian/1 -> MATLAB Function2/1(J)
  weights/1 -> MATLAB Function1/3(weights)
  MATLAB Function2/1(jacobi) -> MATLAB Function1/2(jacobi)
  Constant/1 -> MATLAB Function1/5(jointminvalues)
  Constant1/1 -> MATLAB Function1/6(jointmaxvalues)
  Constant2/1 -> MATLAB Function1/7(joint_min_vel)
  Constant3/1 -> MATLAB Function1/8(joint_max_vel)
  xd_eff_vel/1 -> MATLAB Function1/4(xd_eff_vel)
  Delay/1 -> MATLAB Function1/9(current_joint_vel)
  MATLAB Function1/1(optimal_joint_velocity) -> Scope/1, optimal_joint_velocity/1, Delay/1
  ? -> ?
  ? -> ?
  "b_g "/1 -> MATLAB Function1/11(b_g)
  J_g (distance_Jacobi)/1 -> MATLAB Function1/10(J_g)
  currentconfig/1 -> Transpose/1, Get Jacobian/1
  Transpose/1 -> MATLAB Function1/1(joint_values)

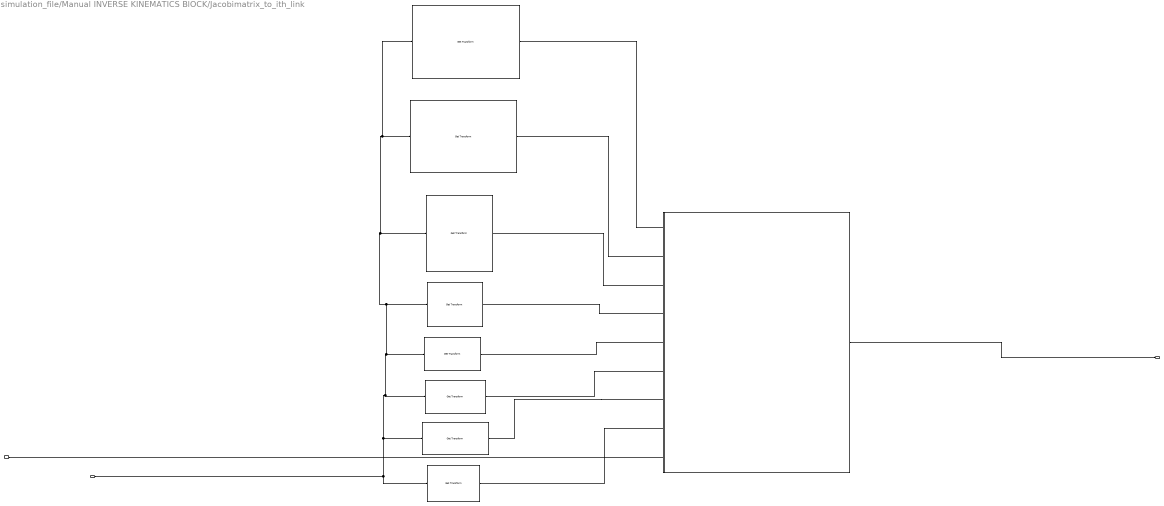
== system simulation_file/Manual INVERSE KINEMATICS BlOCK/Jacobimatrix_to_ith_link ==
  to_ith_link : Inport
  Config : Inport  Port=2
  Get Transform{,1..6} (7 alike) : robotmaniplib/Get Transform  RigidBodyTree=frankarobot_mdh  SourceBody=base  TargetBody=base  SimulateUsing=Interpreted execution
  Get Transform7 : robotmaniplib/Get Transform  RigidBodyTree=frankarobot_mdh  SourceBody=Gripper_TCP  TargetBody=base  SimulateUsing=Interpreted execution
  MATLAB Function : MATLAB Function  TreatAsAtomicUnit=on
  Jacobimatrix : Outport
  wires:
  Get Transform2/1 -> MATLAB Function/5(T05)
  Get Transform3/1 -> MATLAB Function/4(T04)
  Get Transform5/1 -> MATLAB Function/2(T02)
  MATLAB Function/1(Jacobimatrix) -> Jacobimatrix/1
  Get Transform1/1 -> MATLAB Function/6(T06)
  Get Transform/1 -> MATLAB Function/7(T07)
  Get Transform4/1 -> MATLAB Function/3(T03)
  Get Transform6/1 -> MATLAB Function/1(T01)
  Get Transform7/1 -> MATLAB Function/8(T0tcp)
  Config/1 -> Get Transform3/1, Get Transform6/1, Get Transform5/1, Get Transform4/1, Get Transform2/1, Get Transform1/1, Get Transform/1, Get Transform7/1
  to_ith_link/1 -> MATLAB Function/9(to_ith_link)

== system simulation_file/Manual INVERSE KINEMATICS BlOCK/quaternion_error ==
  T : Inport
  In2 : Inport  Port=2
  Enable : EnablePort
  MATLAB Function1 : MATLAB Function  TreatAsAtomicUnit=on
  MATLAB Function2 : MATLAB Function  TreatAsAtomicUnit=on
  Scope : Scope
  Scope1 : Scope
  Transpose1 : Math  Operator=transpose
  qe : Outport
  wires:
  Transpose1/1 -> Scope1/1, MATLAB Function1/1(qd)
  MATLAB Function1/1(qe) -> qe/1
  In2/1 -> Transpose1/1
  MATLAB Function2/1(quat) -> Scope/1, MATLAB Function1/2(qc)
  T/1 -> MATLAB Function1/3(T_i), MATLAB Function2/1(T)

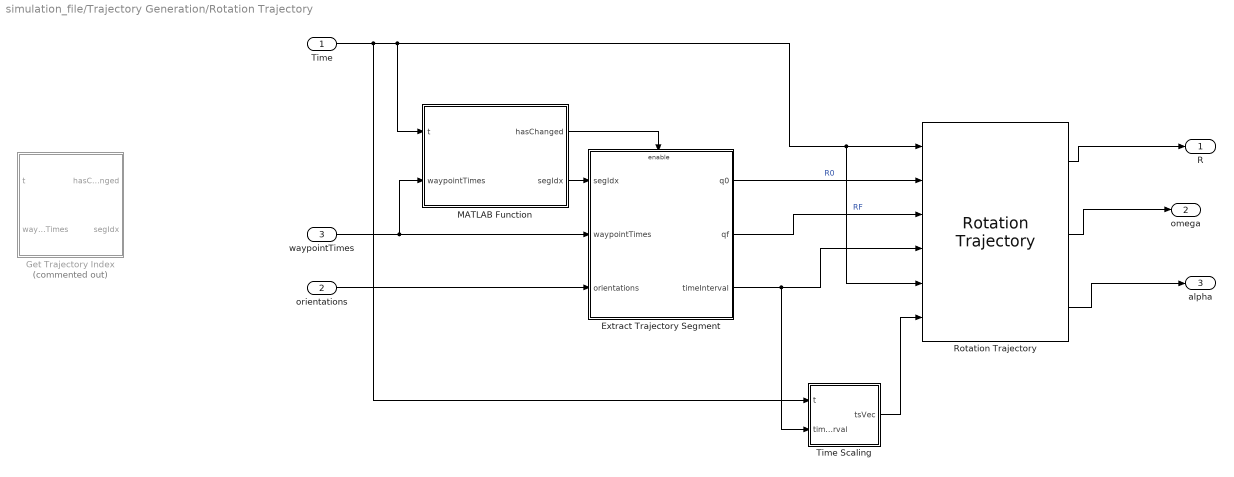
== system simulation_file/Trajectory Generation/Rotation Trajectory ==
  Time : Inport
  orientations : Inport  Port=2
  waypointTimes : Inport  Port=3
  Extract Trajectory Segment : Subsystem
  Get Trajectory Index : MATLAB Function  Commented=on  TreatAsAtomicUnit=on
  MATLAB Function : MATLAB Function  TreatAsAtomicUnit=on
  Rotation Trajectory : robotcorelib/Rotation Trajectory  WaypointFormat=Quaternion  WaypointSource=External  R0=[ 1, 0, 0, 0 ]'  RF=[ 0, 0, 0, 1 ]'  TimeInterval=[ 0, 4 ]  CustomTimeScaling=on  ParameterSource=External  TSTime=0:0.1:1  TimeScaling=[ 0:0.1:1; ones( 1, 11 ); zeros( 1, 11 ) ]  SimulateUsing=Interpreted execution
  Time Scaling : Subsystem
  R : Outport  VectorParamsAs1DForOutWhenUnconnected=off
  omega : Outport  Port=2
  alpha : Outport  Port=3
  wires:
  Rotation Trajectory/1 -> R/1
  Rotation Trajectory/2 -> omega/1
  Rotation Trajectory/3 -> alpha/1
  Extract Trajectory Segment/1(q0) -> Rotation Trajectory/2  "R0"
  Extract Trajectory Segment/2(qf) -> Rotation Trajectory/3  "RF"
  Time/1 -> MATLAB Function/1(t), Rotation Trajectory/5, Rotation Trajectory/1, Time Scaling/1(t)
  waypointTimes/1 -> MATLAB Function/2(waypointTimes), Extract Trajectory Segment/2(waypointTimes)
  MATLAB Function/2(segIdx) -> Extract Trajectory Segment/1(segIdx)
  MATLAB Function/1(hasChanged) -> Extract Trajectory Segment/Enable
  Extract Trajectory Segment/3(timeInterval) -> Time Scaling/2(timeInterval), Rotation Trajectory/4
  orientations/1 -> Extract Trajectory Segment/3(orientations)
  Time Scaling/1(tsVec) -> Rotation Trajectory/6

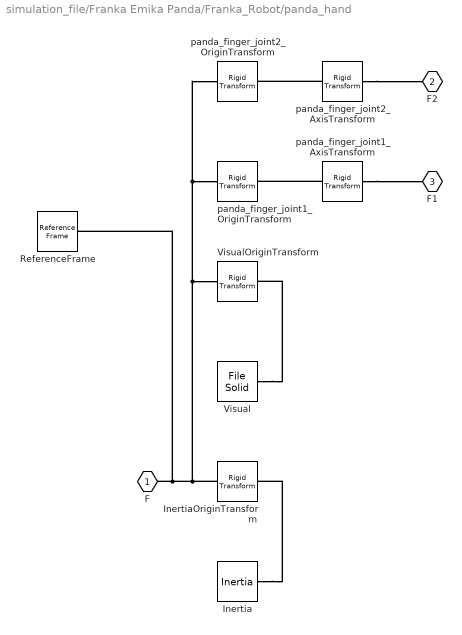
== system simulation_file/Franka Emika Panda/Franka_Robot/panda_hand ==
  Inertia : sm_lib/Body Elements/Inertia  InertiaType=Custom  Mass=0  MassUnits=kg  CenterOfMass=[0, 0, 0]  CenterOfMassUnits=m  MomentsOfInertia=[0, 0, 0]  MomentsOfInertiaUnits=kg*m^2  ProductsOfInertia=[0, 0, 0]  ProductsOfInertiaUnits=kg*m^2  GraphicType=None  MarkerShape=Inertia  MarkerSize=20  GraphicVisPropType=SimpleVisualProperties  GraphicDiffuseColor=[0.5 0.5 0.5]  GraphicSpecularColor=[0.5 0.5 0.5 1.0]  GraphicAmbientColor=[0.15 0.15 0.15 1.0]  GraphicEmissiveColor=[0.0 0.0 0.0 1.0]  GraphicShininess=75  GraphicOpacity=1.0
  InertiaOriginTransform : sm_lib/Frames and Transforms/Rigid Transform  TranslationMethod=Cartesian  TranslationStandardOffset=0  TranslationStandardOffsetUnits=m  TranslationStandardAxis=+Z  TranslationCartesianOffset=[0, 0, 0]  TranslationCartesianOffsetUnits=m  TranslationROffset=0  TranslationROffsetUnits=m  TranslationZOffset=0  TranslationZOffsetUnits=m  TranslationThetaOffset=0  TranslationThetaOffsetUnits=deg  RotationMethod=RotationSequence  RotationAngleUnits=deg  RotationStandardAxis=+Z  RotationAngle=0.0  RotationArbitraryAxis=[0 0 1]  FollAlignAxisA=+X  BaseAlignAxisA=+Y  FollAlignAxisB=+Y  BaseAlignAxisB=+Z  RotationSequenceAxes=BaseAxes  RotationSequence=XYZ  RotationSequenceAngles=[0, 0, 0]  RotationSequenceAnglesUnits=rad  RotationMatrix=[1 0 0; 0 1 0; 0 0 1]  Quaternion=[1 0 0 0]
  ReferenceFrame : sm_lib/Frames and Transforms/Reference Frame
  Visual : sm_lib/Body Elements/File Solid  ExtGeomFileName=/home/shobhit/Documents/MATLAB/SupportPackages/R2023b/toolbox/robotics/supportpackages/robotlibrary/Robots/franka_description/meshes/visual/hand.stl  UnitType=Custom  ExtGeomFileUnits=m  StepReaderType=HEX  ExportConvexHullGeometry=off  InertiaType=Custom  Mass=0  MassUnits=kg  CenterOfMass=[0, 0, 0]  CenterOfMassUnits=m  MomentsOfInertia=[0, 0, 0]  MomentsOfInertiaUnits=kg*m^2  ProductsOfInertia=[0, 0, 0]  ProductsOfInertiaUnits=kg*m^2  BasedOnType=DensityFromFile  Density=1000  DensityUnits=kg/m^3  DoExposeReferenceFrame=on  SerializedFrames=<Frames/>  GraphicType=FromGeometry  MarkerShape=Sphere  MarkerSize=10  GraphicVisPropType=SimpleVisualProperties  GraphicDiffuseColor=[0.5, 0.5, 0.5]  GraphicSpecularColor=[0.5 0.5 0.5 1.0]  GraphicAmbientColor=[0.15 0.15 0.15 1.0]  GraphicEmissiveColor=[0.0 0.0 0.0 1.0]  GraphicShininess=75  GraphicOpacity=1
  VisualOriginTransform : sm_lib/Frames and Transforms/Rigid Transform  TranslationMethod=Cartesian  TranslationStandardOffset=0  TranslationStandardOffsetUnits=m  TranslationStandardAxis=+Z  TranslationCartesianOffset=[0, 0, 0]  TranslationCartesianOffsetUnits=m  TranslationROffset=0  TranslationROffsetUnits=m  TranslationZOffset=0  TranslationZOffsetUnits=m  TranslationThetaOffset=0  TranslationThetaOffsetUnits=deg  RotationMethod=RotationSequence  RotationAngleUnits=deg  RotationStandardAxis=+Z  RotationAngle=0.0  RotationArbitraryAxis=[0 0 1]  FollAlignAxisA=+X  BaseAlignAxisA=+Y  FollAlignAxisB=+Y  BaseAlignAxisB=+Z  RotationSequenceAxes=BaseAxes  RotationSequence=XYZ  RotationSequenceAngles=[0, 0, 0]  RotationSequenceAnglesUnits=rad  RotationMatrix=[1 0 0; 0 1 0; 0 0 1]  Quaternion=[1 0 0 0]
  panda_finger_joint1_AxisTransform : sm_lib/Frames and Transforms/Rigid Transform  TranslationMethod=Cartesian  TranslationStandardOffset=0  TranslationStandardOffsetUnits=m  TranslationStandardAxis=+Z  TranslationCartesianOffset=[0, 0, 0]  TranslationCartesianOffsetUnits=m  TranslationROffset=0  TranslationROffsetUnits=m  TranslationZOffset=0  TranslationZOffsetUnits=m  TranslationThetaOffset=0  TranslationThetaOffsetUnits=deg  RotationMethod=ArbitraryAxis  RotationAngleUnits=rad  RotationStandardAxis=+Z  RotationAngle=1.570796326794897  RotationArbitraryAxis=[-1, 0, 0]  FollAlignAxisA=+X  BaseAlignAxisA=+Y  FollAlignAxisB=+Y  BaseAlignAxisB=+Z  RotationSequenceAxes=FollowerAxes  RotationSequence=XYX  RotationSequenceAngles=[0 0 0]  RotationSequenceAnglesUnits=deg  RotationMatrix=[1 0 0; 0 1 0; 0 0 1]  Quaternion=[1 0 0 0]
  panda_finger_joint1_OriginTransform : sm_lib/Frames and Transforms/Rigid Transform  TranslationMethod=Cartesian  TranslationStandardOffset=0  TranslationStandardOffsetUnits=m  TranslationStandardAxis=+Z  TranslationCartesianOffset=[0, 0, 0.0584]  TranslationCartesianOffsetUnits=m  TranslationROffset=0  TranslationROffsetUnits=m  TranslationZOffset=0  TranslationZOffsetUnits=m  TranslationThetaOffset=0  TranslationThetaOffsetUnits=deg  RotationMethod=RotationSequence  RotationAngleUnits=deg  RotationStandardAxis=+Z  RotationAngle=0.0  RotationArbitraryAxis=[0 0 1]  FollAlignAxisA=+X  BaseAlignAxisA=+Y  FollAlignAxisB=+Y  BaseAlignAxisB=+Z  RotationSequenceAxes=BaseAxes  RotationSequence=XYZ  RotationSequenceAngles=[0, 0, 0]  RotationSequenceAnglesUnits=rad  RotationMatrix=[1 0 0; 0 1 0; 0 0 1]  Quaternion=[1 0 0 0]
  panda_finger_joint2_AxisTransform : sm_lib/Frames and Transforms/Rigid Transform  TranslationMethod=Cartesian  TranslationStandardOffset=0  TranslationStandardOffsetUnits=m  TranslationStandardAxis=+Z  TranslationCartesianOffset=[0, 0, 0]  TranslationCartesianOffsetUnits=m  TranslationROffset=0  TranslationROffsetUnits=m  TranslationZOffset=0  TranslationZOffsetUnits=m  TranslationThetaOffset=0  TranslationThetaOffsetUnits=deg  RotationMethod=ArbitraryAxis  RotationAngleUnits=rad  RotationStandardAxis=+Z  RotationAngle=1.570796326794897  RotationArbitraryAxis=[1, 0, 0]  FollAlignAxisA=+X  BaseAlignAxisA=+Y  FollAlignAxisB=+Y  BaseAlignAxisB=+Z  RotationSequenceAxes=FollowerAxes  RotationSequence=XYX  RotationSequenceAngles=[0 0 0]  RotationSequenceAnglesUnits=deg  RotationMatrix=[1 0 0; 0 1 0; 0 0 1]  Quaternion=[1 0 0 0]
  panda_finger_joint2_OriginTransform : sm_lib/Frames and Transforms/Rigid Transform  TranslationMethod=Cartesian  TranslationStandardOffset=0  TranslationStandardOffsetUnits=m  TranslationStandardAxis=+Z  TranslationCartesianOffset=[0, 0, 0.0584]  TranslationCartesianOffsetUnits=m  TranslationROffset=0  TranslationROffsetUnits=m  TranslationZOffset=0  TranslationZOffsetUnits=m  TranslationThetaOffset=0  TranslationThetaOffsetUnits=deg  RotationMethod=RotationSequence  RotationAngleUnits=deg  RotationStandardAxis=+Z  RotationAngle=0.0  RotationArbitraryAxis=[0 0 1]  FollAlignAxisA=+X  BaseAlignAxisA=+Y  FollAlignAxisB=+Y  BaseAlignAxisB=+Z  RotationSequenceAxes=BaseAxes  RotationSequence=XYZ  RotationSequenceAngles=[0, 0, 0]  RotationSequenceAnglesUnits=rad  RotationMatrix=[1 0 0; 0 1 0; 0 0 1]  Quaternion=[1 0 0 0]
  F : PMIOPort  Side=Left
  F2 : PMIOPort  Port=2  Side=Right
  F1 : PMIOPort  Port=3  Side=Right
  connections:
  Inertia/RConn1 -- InertiaOriginTransform/RConn1
  ReferenceFrame/RConn1 -- InertiaOriginTransform/LConn1 -- panda_finger_joint1_OriginTransform/LConn1 -- panda_finger_joint2_OriginTransform/LConn1 -- VisualOriginTransform/LConn1 -- F/RConn1
  Visual/RConn1 -- VisualOriginTransform/RConn1
  panda_finger_joint1_AxisTransform/RConn1 -- F1/RConn1
  panda_finger_joint1_AxisTransform/LConn1 -- panda_finger_joint1_OriginTransform/RConn1
  panda_finger_joint2_AxisTransform/RConn1 -- F2/RConn1
  panda_finger_joint2_AxisTransform/LConn1 -- panda_finger_joint2_OriginTransform/RConn1
